simulink model "Q4"  (R2018a)
settings: Solver=VariableStepAuto  StartTime=0.0  StopTime=10  FixedStep=0.01  RelTol=1e-3
settings Model: Creator=Halil Temurtaş  LastModifiedBy=Halil Temurtaş

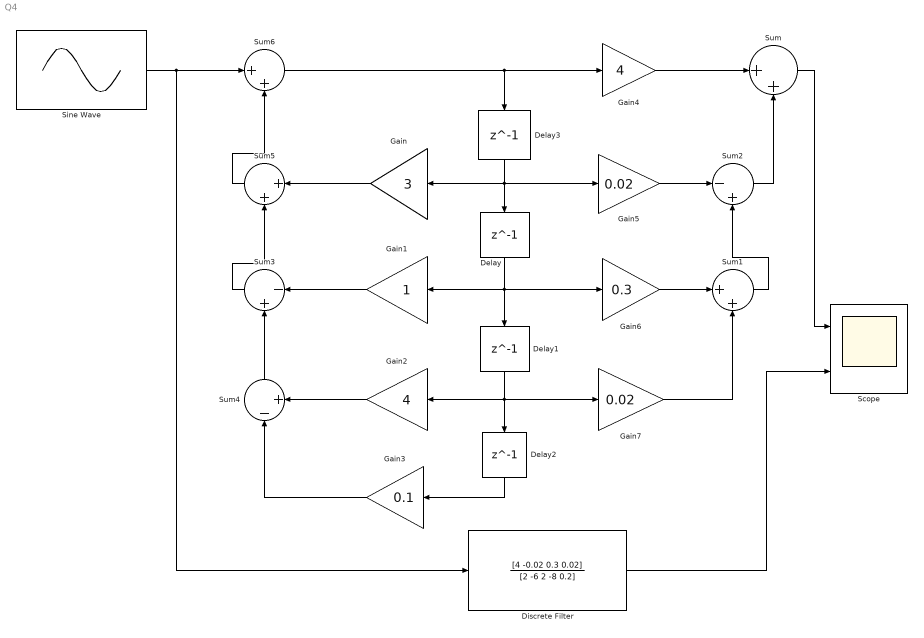
== system Q4 ==
  Delay{,1..3} (4 alike) : Delay  DelayLength=1
  Discrete Filter : DiscreteFilter  Numerator=[4 -0.02 0.3 0.02]  Denominator=[2 -6 2 -8 0.2]
  Gain : Gain  Gain=3
  Gain1 : Gain
  Gain2 : Gain  Gain=4
  Gain3 : Gain  Gain=0.1
  Gain4 : Gain  Gain=4
  Gain5 : Gain  Gain=0.02
  Gain6 : Gain  Gain=0.3
  Gain7 : Gain  Gain=0.02
  Scope : Scope  NumInputPorts=2
  Sine Wave : Sin  Frequency=10  SampleTime=0
  Sum{,1,5..6} (4 alike) : Sum  Inputs=|++
  Sum2 : Sum  Inputs=|-+
  Sum3 : Sum  Inputs=|-+
  Sum4 : Sum  Inputs=|-+
  wires:
  Delay/1 -> Gain6/1, Delay1/1, Gain1/1
  Delay1/1 -> Gain7/1, Delay2/1, Gain2/1
  Delay3/1 -> Gain5/1, Delay/1, Gain/1
  Delay2/1 -> Gain3/1
  Gain4/1 -> Sum/1
  Sum2/1 -> Sum/2
  Gain6/1 -> Sum1/1
  Gain7/1 -> Sum1/2
  Gain5/1 -> Sum2/1
  Sum1/1 -> Sum2/2
  Gain3/1 -> Sum4/1
  Sum4/1 -> Sum3/2
  Gain2/1 -> Sum4/2
  Gain1/1 -> Sum3/1
  Gain/1 -> Sum5/1
  Sum3/1 -> Sum5/2
  Sum/1 -> Scope/1
  Sum5/1 -> Sum6/2
  Sum6/1 -> Gain4/1, Delay3/1
  Sine Wave/1 -> Discrete Filter/1, Sum6/1
  Discrete Filter/1 -> Scope/2
